simulink model "CarlaRosMatlab_KeyboardControl"  (R2019b)
settings: Solver=FixedStepAuto  StartTime=0.0  StopTime=inf  FixedStep=0.2  RelTol=1e-3  EnableMultiTasking=on
model workspace (MAT data in the model file):
  SL_ROS_VariableLengthArrays_MaxSizes.CommonInfo.ArrayTruncateAction = 'EmitWarning'
  SL_ROS_VariableLengthArrays_MaxSizes.MsgTypeMap = containers.Map
  SL_ROS_VariableLengthArrays_MaxSizes.MsgTypeMap.serialization.keys = {'sensor_msgs/CompressedImage', 'sensor_msgs/Image', 'sensor_msgs/PointCloud2'}
  SL_ROS_VariableLengthArrays_MaxSizes.MsgTypeMap.serialization.values{1}(1).PropertyName = 'Format'
  SL_ROS_VariableLengthArrays_MaxSizes.MsgTypeMap.serialization.values{1}(1).DataType = 'uint8'
  SL_ROS_VariableLengthArrays_MaxSizes.MsgTypeMap.serialization.values{1}(1).MaxLength = 128
  SL_ROS_VariableLengthArrays_MaxSizes.MsgTypeMap.serialization.values{1}(2).PropertyName = 'Data'
  SL_ROS_VariableLengthArrays_MaxSizes.MsgTypeMap.serialization.values{1}(2).DataType = 'uint8'
  SL_ROS_VariableLengthArrays_MaxSizes.MsgTypeMap.serialization.values{1}(2).MaxLength = 128000
  SL_ROS_VariableLengthArrays_MaxSizes.MsgTypeMap.serialization.values{2}(1).PropertyName = 'Data'
  SL_ROS_VariableLengthArrays_MaxSizes.MsgTypeMap.serialization.values{2}(1).DataType = 'uint8'
  SL_ROS_VariableLengthArrays_MaxSizes.MsgTypeMap.serialization.values{2}(1).MaxLength = 3686400
  SL_ROS_VariableLengthArrays_MaxSizes.MsgTypeMap.serialization.values{2}(2).PropertyName = 'Encoding'
  SL_ROS_VariableLengthArrays_MaxSizes.MsgTypeMap.serialization.values{2}(2).DataType = 'uint8'
  SL_ROS_VariableLengthArrays_MaxSizes.MsgTypeMap.serialization.values{2}(2).MaxLength = 128
  SL_ROS_VariableLengthArrays_MaxSizes.MsgTypeMap.serialization.values{3}(1).PropertyName = 'Data'
  SL_ROS_VariableLengthArrays_MaxSizes.MsgTypeMap.serialization.values{3}(1).DataType = 'uint8'
  SL_ROS_VariableLengthArrays_MaxSizes.MsgTypeMap.serialization.values{3}(1).MaxLength = 179160
  SL_ROS_VariableLengthArrays_MaxSizes.MsgTypeMap.serialization.values{3}(2).PropertyName = 'Fields'
  SL_ROS_VariableLengthArrays_MaxSizes.MsgTypeMap.serialization.values{3}(2).DataType = 'sensor_msgs/PointField'
  SL_ROS_VariableLengthArrays_MaxSizes.MsgTypeMap.serialization.values{3}(2).MaxLength = 16
  SL_ROS_VariableLengthArrays_MaxSizes.MsgTypeMap.serialization.uniformity = 0
  SL_ROS_VariableLengthArrays_MaxSizes.MsgTypeMap.serialization.keyType = 'char'
  SL_ROS_VariableLengthArrays_MaxSizes.MsgTypeMap.serialization.valueType = 'any'
undefined symbols (not defined in the file or in its folder): Brake, Reverse, Steer, Throttle
libraries: robotlib x8, visionsinks x2, visiontextngfix x1
settings Model: Creator=sprinkle  LastModifiedBy=aa
settings DataIOCC: ReturnWorkspaceOutputs=off
settings OptimizationCC: LifeSpan=Inf  MaxStackSize=64  EfficientTunableParamExpr=on
settings DebuggingCC: SFUnexpectedBacktrackingDiag=warning  SFNoUnconditionalDefaultTransitionDiag=warning  ArithmeticOperatorsInVariantConditions=warning
settings HardwareCC: ProdBitPerPointer=32  ProdBitPerSizeT=32  ProdBitPerPtrDiffT=32  ProdLargestAtomicFloat=None  ProdIntDivRoundTo=Undefined  ProdEndianess=Unspecified  ProdWordSize=32  ProdHWDeviceType=Generic->Unspecified (assume 32-bit Generic)
settings SFSimCC: SimUseLocalCustomCode=off  MATLABDynamicMemAlloc=off  CustomCodeUndefinedFunction=UseInterfaceOnly
settings RTWCC: SystemTargetFile=ert.tlc  HardwareBoard=Robot Operating System (ROS)  TLCOptions=-aInlineSetEventsForThisBaseRateFcn=TLC_FALSE -aSuppressMultiTaskScheduler=TLC_FALSE -aRateBasedStepFcn=0  TemplateMakefile=ert_default_tmf  GenerateReport=on  RTWUseLocalCustomCode=off  Toolchain=Catkin  IncludeHyperlinkInReport=on  LaunchReport=on  TargetLang=C++  GenerateTraceInfo=on  GenerateTraceReport=on  GenerateTraceReportSl=on  GenerateTraceReportSf=on  GenerateTraceReportEml=on
settings CodeAppCC: ForceParamTrailComments=on  IgnoreCustomStorageClasses=off  OperatorAnnotations=on  SimulinkDataObjDesc=on  SFDataObjDesc=on  MATLABFcnDesc=on  InsertBlockDesc=on  StateflowObjectComments=on  MATLABSourceComments=on
settings ERTTargetCC: MultiwordLength=2048
settings ConfigComp: CovMetricSettings=dw  CovHtmlReporting=on  CovSaveCumulativeToWorkspaceVar=on  CovSaveSingleToWorkspaceVar=on  CovExternalEMLEnable=off

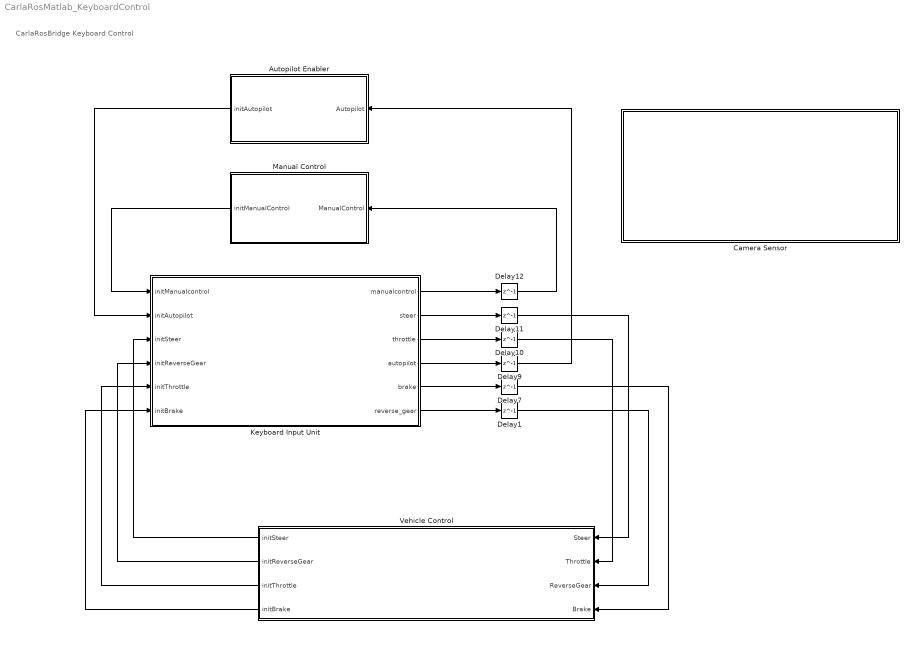
== system CarlaRosMatlab_KeyboardControl ==
  note: CarlaRosBridge Keyboard Control
  Autopilot Enabler : Subsystem
  Camera Sensor : Subsystem
  Delay{1,7,9..12} (6 alike) : Delay  DelayLength=1  InitialCondition=0
  Keyboard Input Unit : Subsystem
  Manual Control : Subsystem
  Vehicle Control : Subsystem
  wires:
  Delay11/1 -> Vehicle Control/1(Steer)
  Delay10/1 -> Vehicle Control/2(Throttle)
  Delay7/1 -> Vehicle Control/4(Brake)
  Delay9/1 -> Autopilot Enabler/1(Autopilot)
  Autopilot Enabler/1(initAutopilot) -> Keyboard Input Unit/2(initAutopilot)
  Vehicle Control/1(initSteer) -> Keyboard Input Unit/3(initSteer)
  Vehicle Control/2(initReverseGear) -> Keyboard Input Unit/4(initReverseGear)
  Vehicle Control/3(initThrottle) -> Keyboard Input Unit/5(initThrottle)
  Vehicle Control/4(initBrake) -> Keyboard Input Unit/6(initBrake)
  Keyboard Input Unit/1(manualcontrol) -> Delay12/1
  Keyboard Input Unit/2(steer) -> Delay11/1
  Keyboard Input Unit/3(throttle) -> Delay10/1
  Keyboard Input Unit/4(autopilot) -> Delay9/1
  Keyboard Input Unit/5(brake) -> Delay7/1
  Keyboard Input Unit/6(reverse_gear) -> Delay1/1
  Delay12/1 -> Manual Control/1(ManualControl)
  Manual Control/1(initManualControl) -> Keyboard Input Unit/1(initManualcontrol)
  Delay1/1 -> Vehicle Control/3(ReverseGear)

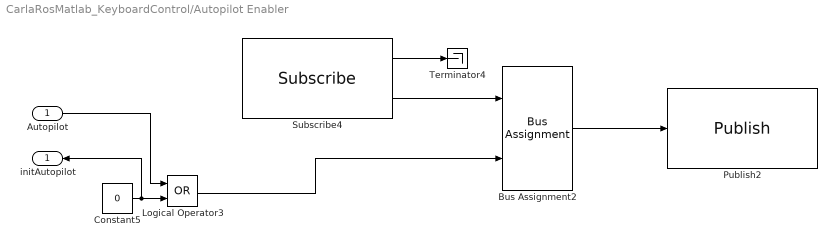
== system CarlaRosMatlab_KeyboardControl/Autopilot Enabler ==
  Autopilot : Inport
  Bus Assignment2 : BusAssignment  AssignedSignals=Data
  Constant5 : Constant  Value=0  OutDataTypeStr=boolean
  Logical Operator3 : Logic  Operator=OR  AllPortsSameDT=off  OutDataTypeStr=boolean
  Publish2 : robotlib/Publish  topicSource=Select from ROS network  topic=/carla/ego_vehicle/enable_autopilot  messageType=std_msgs/Bool  messageQueueLength=1
      settings: SourceProductName=ROS Toolbox
  Subscribe4 : robotlib/Subscribe  topicSource=Select from ROS network  topic=/carla/ego_vehicle/enable_autopilot  messageType=std_msgs/Bool  sampleTime=-1  messageQueueLength=1
      settings: SourceProductName=ROS Toolbox
  Terminator4 : Terminator
  initAutopilot : Outport
  wires:
  Logical Operator3/1 -> Bus Assignment2/2
  Autopilot/1 -> Logical Operator3/1
  Bus Assignment2/1 -> Publish2/1
  Subscribe4/1 -> Terminator4/1
  Constant5/1 -> Logical Operator3/2, initAutopilot/1
  Subscribe4/2 -> Bus Assignment2/1

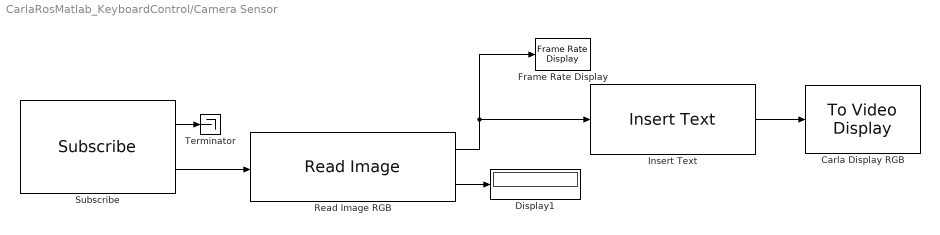
== system CarlaRosMatlab_KeyboardControl/Camera Sensor ==
  Carla Display RGB : visionsinks/To Video Display  windowSizeMode=Normal  openAtMdlStart=on  fullScreen=off  videoWindowX=307  videoWindowY=85  saveWindowSize=off  videoWindowWidth=551  videoWindowHeight=468  inputColorFormat=RGB  inputType=Obsolete  imagePorts=One multidimensional signal  OutputDevice=On-screen video monitor  dataOrg=Column-major  isWindowOpen=off
      settings: SourceProductName=Computer Vision Toolbox
  Display1 : Display
  Frame Rate Display : visionsinks/Frame Rate Display  UpdateRate=10
      settings: SourceProductName=Computer Vision Toolbox  SourceProductBaseCode=VP
  Insert Text : visiontextngfix/Insert Text  inputType=Obsolete  theText='Carla Ros Bridge RGB Camera'  getTextLocFrom=Specify via dialog  textLoc=[1 1]  getTextColorFrom=Specify via dialog  textColor=[0 0 0]  getTextIntensityFrom=Specify via dialog  textIntensity=0  getTextOpacityFrom=Specify via dialog  textOpacity=1.0  dummyVar2=0  dummyVar3=0  dummyVar4=0  imagePorts=One multidimensional signal  isInputTransposed=off  fontFace=LucidaSansRegular  dummyVar1=0  blockFontSize=24  antiAliased=on
      settings: SourceProductName=Computer Vision Toolbox  SourceProductBaseCode=VP
  Read Image RGB : robotlib/Read Image  MaximumImageSize=[600, 800]  ImageEncoding=bgra8  ShowAlphaOutput=off  ShowErrorCodeOutput=on  VariableSizeOutputs=on
      settings: SourceProductName=Robotics System Toolbox  SourceProductBaseCode=RO
  Subscribe : robotlib/Subscribe  topicSource=Select from ROS network  topic=/carla/ego_vehicle/camera/rgb/front/image_color  messageType=sensor_msgs/Image  sampleTime=-1  messageQueueLength=1
      settings: SourceProductBaseCode=RO
  Terminator : Terminator
  wires:
  Subscribe/2 -> Read Image RGB/1
  Read Image RGB/1 -> Frame Rate Display/1, Insert Text/1
  Subscribe/1 -> Terminator/1
  Read Image RGB/2 -> Display1/1
  Insert Text/1 -> Carla Display RGB/1

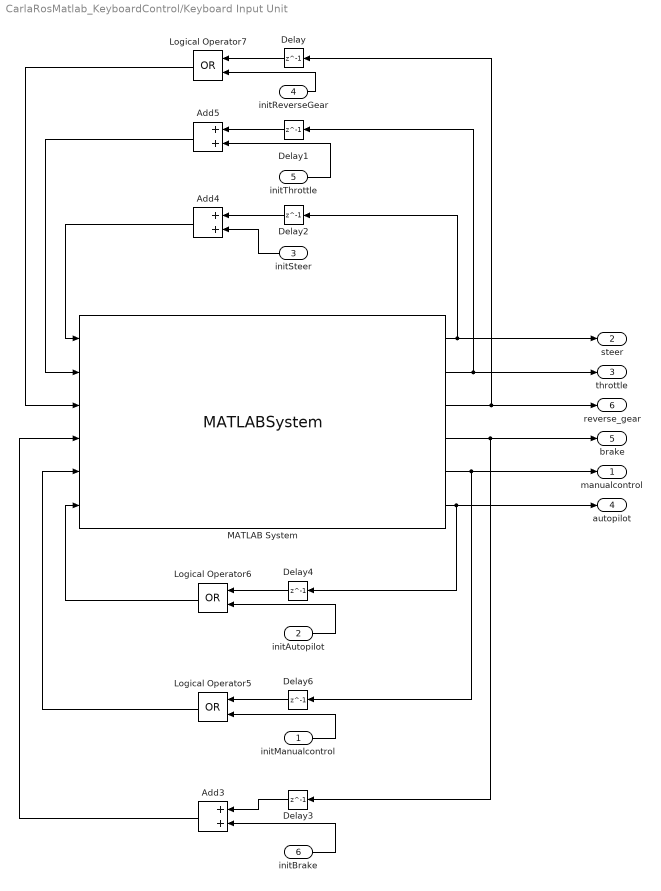
== system CarlaRosMatlab_KeyboardControl/Keyboard Input Unit ==
  initManualcontrol : Inport
  initAutopilot : Inport  Port=2
  initSteer : Inport  Port=3
  initReverseGear : Inport  Port=4
  initThrottle : Inport  Port=5
  initBrake : Inport  Port=6
  Add3 : Sum
  Add4 : Sum
  Add5 : Sum
  Delay{,1..4,6} (6 alike) : Delay  DelayLength=1  InitialCondition=0
  Logical Operator5 : Logic  Operator=OR  AllPortsSameDT=off  OutDataTypeStr=boolean
  Logical Operator6 : Logic  Operator=OR  AllPortsSameDT=off  OutDataTypeStr=boolean
  Logical Operator7 : Logic  Operator=OR  AllPortsSameDT=off  OutDataTypeStr=boolean
  MATLAB System : MATLABSystem  System=KeyboardControl  SimulateUsing=Interpreted execution
      mask Type: KeyboardControl
      mask Display:
      | disp('KeyboardControl');
      | port_label('input',1,'steer_prev');
      | port_label('input',2,'throttle_prev');
      | port_label('input',3,'reverse_gear_prev');
      | port_label('input',4,'brake_prev');
      | port_label('input',5,'manualcontrol_prev');
      | port_label('input',6,'autopilot_prev');
      | port_label('output',1,'steer');
      | port_label('output',2,'throttle');
      | port_label('output',3,'reverse_gear');
      | port_label('output',4,'brake');
      | port_label('output',5,'manualcontrol');
      | port_label('output',6,'autopilot');
  manualcontrol : Outport
  steer : Outport  Port=2
  throttle : Outport  Port=3
  autopilot : Outport  Port=4
  brake : Outport  Port=5
  reverse_gear : Outport  Port=6
  wires:
  initAutopilot/1 -> Logical Operator6/2
  Delay1/1 -> Add5/1
  Delay/1 -> Logical Operator7/1
  initManualcontrol/1 -> Logical Operator5/2
  Add5/1 -> MATLAB System/2
  MATLAB System/2 -> throttle/1, Delay1/1
  MATLAB System/6 -> Delay4/1, autopilot/1
  MATLAB System/4 -> brake/1, Delay3/1
  MATLAB System/5 -> manualcontrol/1, Delay6/1
  MATLAB System/3 -> Delay/1, reverse_gear/1
  MATLAB System/1 -> Delay2/1, steer/1
  Logical Operator7/1 -> MATLAB System/3
  Logical Operator5/1 -> MATLAB System/5
  Delay6/1 -> Logical Operator5/1
  initThrottle/1 -> Add5/2
  initSteer/1 -> Add4/2
  Add3/1 -> MATLAB System/4
  Logical Operator6/1 -> MATLAB System/6
  Delay4/1 -> Logical Operator6/1
  Delay2/1 -> Add4/1
  initReverseGear/1 -> Logical Operator7/2
  Add4/1 -> MATLAB System/1
  Delay3/1 -> Add3/1
  initBrake/1 -> Add3/2

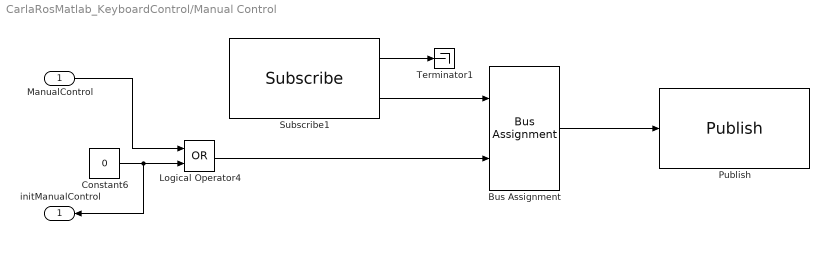
== system CarlaRosMatlab_KeyboardControl/Manual Control ==
  ManualControl : Inport
  Bus Assignment : BusAssignment  AssignedSignals=Data
  Constant6 : Constant  Value=0  OutDataTypeStr=boolean
  Logical Operator4 : Logic  Operator=OR  AllPortsSameDT=off  OutDataTypeStr=boolean
  Publish : robotlib/Publish  topicSource=Select from ROS network  topic=/carla/ego_vehicle/vehicle_control_manual_override  messageType=std_msgs/Bool  messageQueueLength=1
      settings: SourceProductName=ROS Toolbox
  Subscribe1 : robotlib/Subscribe  topicSource=Select from ROS network  topic=/carla/ego_vehicle/vehicle_control_manual_override  messageType=std_msgs/Bool  sampleTime=-1  messageQueueLength=1
      settings: SourceProductName=ROS Toolbox
  Terminator1 : Terminator
  initManualControl : Outport
  wires:
  Constant6/1 -> Logical Operator4/2, initManualControl/1
  Subscribe1/1 -> Terminator1/1
  Logical Operator4/1 -> Bus Assignment/2
  ManualControl/1 -> Logical Operator4/1
  Bus Assignment/1 -> Publish/1
  Subscribe1/2 -> Bus Assignment/1

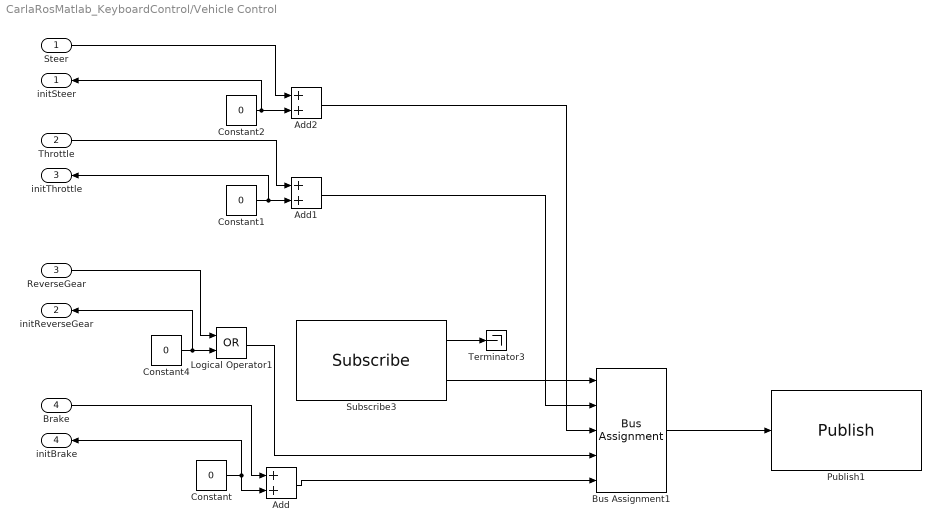
== system CarlaRosMatlab_KeyboardControl/Vehicle Control ==
  Steer : Inport
  Throttle : Inport  Port=2
  ReverseGear : Inport  Port=3
  Brake : Inport  Port=4
  Add : Sum
  Add1 : Sum
  Add2 : Sum
  Bus Assignment1 : BusAssignment  AssignedSignals=Throttle,Steer,Reverse,Brake
  Constant : Constant  Value=0  OutDataTypeStr=single
  Constant1 : Constant  Value=0  OutDataTypeStr=single
  Constant2 : Constant  Value=0  OutDataTypeStr=single
  Constant4 : Constant  Value=0  OutDataTypeStr=boolean
  Logical Operator1 : Logic  Operator=OR  AllPortsSameDT=off  OutDataTypeStr=boolean
  Publish1 : robotlib/Publish  topicSource=Select from ROS network  topic=/carla/ego_vehicle/vehicle_control_cmd_manual  messageType=carla_msgs/CarlaEgoVehicleControl  messageQueueLength=1
      settings: SourceProductName=ROS Toolbox
  Subscribe3 : robotlib/Subscribe  topicSource=Select from ROS network  topic=/carla/ego_vehicle/vehicle_control_cmd_manual  messageType=carla_msgs/CarlaEgoVehicleControl  sampleTime=-1  messageQueueLength=1
      settings: SourceProductName=ROS Toolbox
  Terminator3 : Terminator
  initSteer : Outport
  initReverseGear : Outport  Port=2
  initThrottle : Outport  Port=3
  initBrake : Outport  Port=4
  wires:
  Steer/1 -> Add2/1
  Constant2/1 -> initSteer/1, Add2/2
  ReverseGear/1 -> Logical Operator1/1
  Throttle/1 -> Add1/1
  Constant1/1 -> initThrottle/1, Add1/2
  Constant/1 -> initBrake/1, Add/2
  Constant4/1 -> Logical Operator1/2, initReverseGear/1
  Brake/1 -> Add/1
  Add1/1 -> Bus Assignment1/2
  Subscribe3/1 -> Terminator3/1
  Subscribe3/2 -> Bus Assignment1/1
  Add2/1 -> Bus Assignment1/3
  Bus Assignment1/1 -> Publish1/1
  Logical Operator1/1 -> Bus Assignment1/4
  Add/1 -> Bus Assignment1/5
